simulink model "c6713dskfblms"  (Simulink 6.0)
settings: Solver=FixedStepDiscrete  StartTime=0.0  StopTime=inf  RelTol=1e-3
PreLoadFcn:
  | load handel; audiofrag = int16(y(1:2^16).*2^14); clear y;
undefined symbols (not defined in the file or in its folder): bit, FFT, FixedBlocks, Norm
libraries: tic62dsplib x17, dspmtrx3 x5, simulink x4, c6713dsklib x3, dspsnks4 x3, dspsigops x2, c6000tgtpreflib x1, dspbuff3 x1, dspxfrm3 x1, dspsrcs4 x1
settings Model: Creator=adowd  LastModifiedBy=thartley  ProdHWDeviceType=TI C6000
settings DataIOCC: SaveOutput=off  SaveTime=off  SignalLoggingName=sigsOut
settings OptimizationCC: InlineInvariantSignals=off  LocalBlockOutputs=off
settings DebuggingCC: CheckExecutionContextPreStartOutputMsg=on  CheckExecutionContextRuntimeOutputMsg=on  SolverPrmCheckMsg=none  IntegerOverflowMsg=none  ParameterPrecisionLossMsg=none
settings HardwareCC: ProdBitPerLong=40  ProdEndianess=LittleEndian  ProdHWDeviceType=TI C6000  TargetHWDeviceType=32-bit Generic
settings ModelReferenceCC: UpdateModelReferenceTargets=IfOutOfDate
settings RTWCC: SystemTargetFile=ti_c6000.tlc  GenCodeOnly=on  TemplateMakefile=ti_c6000.tmf  ProcessScript=ti_c6000_make_rtw_hook
settings CodeAppCC: PrefixModelToSubsysFcnNames=off
settings STFCustomTargetCC: TargetFcnLib=ansi_tfl_tmw.mat  GenFloatMathFcnCalls=ANSI_C  ModelReferenceCompliant=off  SystemTargetFile=ti_c6000.tlc  ActivateCallback=c6000_callback('ActivateCallback',hSrc,hDlg);  ForcedBaseTarget=off
settings GRTTargetCC: ModelReferenceCompliant=off  MatFileLogging=off
settings CustomProperty: DataType=RTWOptions_EnumType_s__Adsphw_matlab_toolbox_rtw_targets_tic6000_tic6000_ti_c6000_BoardType  Value=C6713DSK
settings EnumStrPairs: String=C6416DSK
settings SFSimCC: SFSimApplyToAllLibs=on  SFSimBuildMode=Incremental

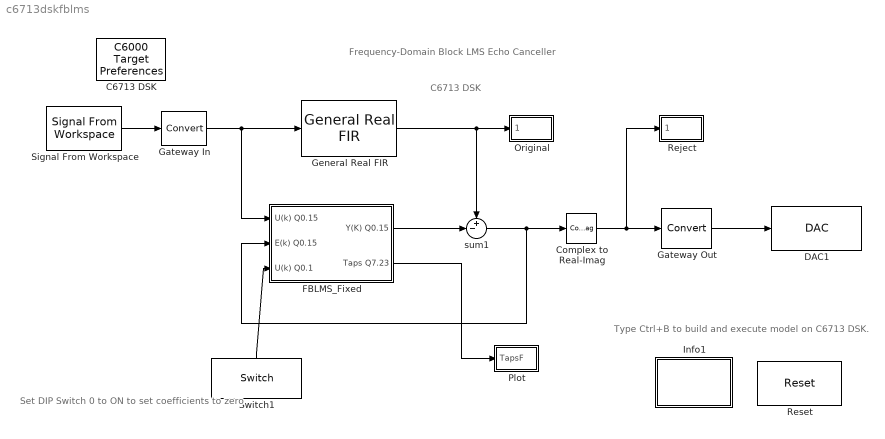
== system c6713dskfblms ==
  note: Frequency-Domain Block LMS
      | Echo Canceller
  note: Type Ctrl+B to build
      | and execute model
      | on C6713 DSK.
  note: C6713 DSK
  note: Set DIP Switch 0 to ON
      | to set coefficients to zero
  C6713 DSK : c6000tgtpreflib/C6000 Target Preferences
  Complex to Real-Imag : ComplexToRealImag  Output=Real
  DAC1 : c6713dsklib/DAC  CodecDataFormat=16-bit  Scaling=Integer Value  DacAtten=0.0  OverflowMode=Saturate
  FBLMS_Fixed : Subsystem  PropExecContextAcrossSSBoundary=on
  Gateway In : DataTypeConversion  OutDataTypeMode=Specify via dialog  OutDataType=sfrac(16)  OutScaling=2^-10  ConvertRealWorld=Stored Integer (SI)
  Gateway Out : DataTypeConversion  OutDataTypeMode=int16  ConvertRealWorld=Stored Integer (SI)
  General Real FIR : tic62dsplib/General Real FIR  coeff_source=Specify via dialog  coeffs=fir1(63,0.25)  ic_arg=0
  Info1 : Subsystem  PropExecContextAcrossSSBoundary=on
      settings: OpenFcn=web(fullfile(matlabroot,'toolbox','rtw','targets','tic6000','tic6000demos','html','fblms_doc.html'))
      mask Type: Frame-Based Simulation Info
      mask Display: disp('Info')
  Original : Subsystem  TreatAsAtomicUnit=on  PropExecContextAcrossSSBoundary=on  SimViewingDevice=on
  Plot : Subsystem  TreatAsAtomicUnit=on  PropExecContextAcrossSSBoundary=on  SimViewingDevice=on
  Reject : Subsystem  TreatAsAtomicUnit=on  PropExecContextAcrossSSBoundary=on  SimViewingDevice=on
  Reset : c6713dsklib/Reset
  Signal From Workspace : dspsrcs4/Signal From Workspace  X=audiofrag  Ts=1/8000  nsamps=64  OutputAfterFinalValue=Cyclic repetition
  Switch1 : c6713dsklib/Switch  Orientation=up  sw0=off  sw1=off  sw2=off  sw3=off  dType=Boolean  Ts=64/8000
  sum1 : Sum  Inputs=+-|  SaturateOnIntegerOverflow=on  InputSameDT=on
  wires:
  FBLMS_Fixed/1(Y(K) Q0.15) -> sum1/2
  General Real FIR/1 -> sum1/1, Original/1(Signal)
  Complex to Real-Imag/1 -> Gateway Out/1, Reject/1(Signal)
  Gateway Out/1 -> DAC1/1
  sum1/1 -> FBLMS_Fixed/2(E(k) Q0.15), Complex to Real-Imag/1
  Gateway In/1 -> General Real FIR/1, FBLMS_Fixed/1(U(k) Q0.15)
  FBLMS_Fixed/2(Taps Q7.23) -> Plot/1(TapsF)
  Signal From Workspace/1 -> Gateway In/1
  Switch1/1 -> FBLMS_Fixed/3(U(k) Q0.1)

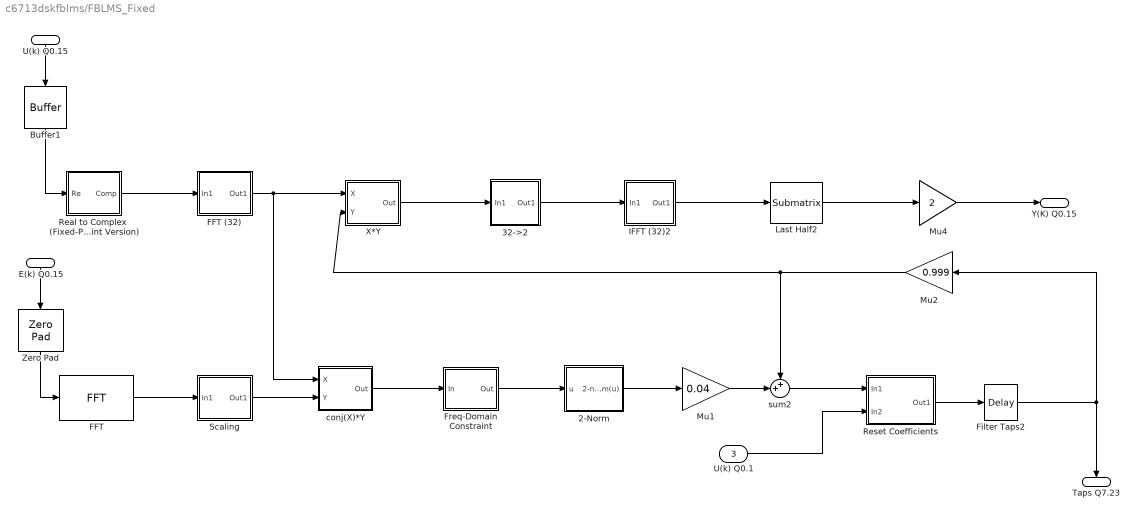
== system c6713dskfblms/FBLMS_Fixed ==
  U(k) Q0.15 : Inport  Orientation=down  LatchInput=off
  E(k) Q0.15 : Inport  Orientation=down  Port=2  LatchInput=off
  U(k) Q0.1 : Inport  Port=3  LatchInput=off
  2-Norm : Subsystem  AncestorBlock=FixedBlocks/2-Norm  PropExecContextAcrossSSBoundary=on
  32->2 : Subsystem  PropExecContextAcrossSSBoundary=on
  Buffer1 : dspbuff3/Buffer  Orientation=down  N=128  V=64  ic=0
  FFT : tic62dsplib/FFT
  FFT (32) : Subsystem  AncestorBlock=FixedBlocks/FFT (32)  PropExecContextAcrossSSBoundary=on  mask{nlen=128, prescale=1/4, postscale=32}
      mask prompts: nlen "Length (8 to 16384)"; prescale "Prescaling (8:32->1/4, 64:512->1/8)"; postscale "Postscaling"
      mask help:
      | This block performs an IFFT with output returned in normal (NOT bit-reversed order).
      | The implemented uses the FFT block.  This includes some scaling to avoid overflow
      | AND some scaling to compensate for scaling factors in FFT16X16R block
      mask CallbackString:
      | x = get_param(gcb,'MaskValues');
      | tscale = [2 2 4 4 8 8 16 16 32 32];
      | indx = round(log(eval(x{1}))/log(2)-2);
      | scale = tscale(indx);
      | x{3} = num2str(scale/eval(x{2}));
      | set_param(gcb,'MaskValues',x);|x = get_param(gcb,'MaskValues');
      | tscale = [2 2 4 4 8 8 16 16 32 32];
      | indx = round(log(eval(x{1}))/log(2)-2);
      | scale = tscale(indx);
      | x{3} = num2str(scale/eval(x{2}));
      | set_param(gcb,'MaskValues',x);|
  Filter Taps2 : dspsigops/Delay  dly_unit=Samples  delay=1  ic_detail=off  dif_ic_for_ch=off  dif_ic_for_dly=off  ic=0  reset_popup=None
  Freq-Domain Constraint : Subsystem  PropExecContextAcrossSSBoundary=on
  IFFT (32)2 : Subsystem  PropExecContextAcrossSSBoundary=on  mask{nlen=128, prescale=1/2, postscale=0.125}
      mask prompts: nlen "Length (8 to 16384)"; prescale "Prescaling"; postscale "Postscaling"
      mask init:
      | scale = 2.^(floor(log(nlen)/log(4))+1);
      | postscale = 1/(scale*prescale);
      mask CallbackString:
      | x = get_param(gcb,'MaskValues');
      | scale = 2.^(floor(log(eval(x{1}))/log(4))+1);
      | x{3} = num2str(1/(scale*eval(x{2})));
      | set_param(gcb,'MaskValues',x);|x = get_param(gcb,'MaskValues');
      | scale = 2.^(floor(log(eval(x{1}))/log(4))+1);
      | x{3} = num2str(1/(scale*eval(x{2})));
      | set_param(gcb,'MaskValues',x);|
  Last Half2 : dspmtrx3/Submatrix  RowSpan=Range of rows  RowStartMode=Offset from middle  RowStartIndex=0  RowEndMode=Last  RowEndIndex=L  ColSpan=All columns  ColStartMode=First  ColStartIndex=1  ColEndMode=Last  ColEndIndex=1
  Mu1 : Gain  Gain=0.04  OutDataTypeMode=Specify via dialog  OutDataType=sfix(32)  OutScaling=2^-31
  Mu2 : Gain  Orientation=left  Gain=0.999  SaturateOnIntegerOverflow=on
  Mu4 : Gain  Gain=2  SaturateOnIntegerOverflow=on
  Real to Complex  (Fixed-Point Version) : Subsystem  PropExecContextAcrossSSBoundary=on
  Reset Coefficients : Subsystem  PropExecContextAcrossSSBoundary=on
  Scaling : Subsystem  PropExecContextAcrossSSBoundary=on
  X*Y : Subsystem  PropExecContextAcrossSSBoundary=on
  Zero Pad : dspsigops/Zero Pad  Orientation=down  padSigAt=Beginning  zpadAlong=Columns  padNumOutRowsSpecMethod=User-specified  numOutRows=128  padNumOutColsSpecMethod=Next power of two  numOutCols=1  trunc_flag=None
      settings: AttributesFormatString=\n
  conj(X)*Y : Subsystem  PropExecContextAcrossSSBoundary=on
  sum2 : Sum  Inputs=++|  OutDataTypeMode=Specify via dialog  OutDataType=sfix(32)  OutScaling=2^-24  SaturateOnIntegerOverflow=on
  Y(K) Q0.15 : Outport
  Taps Q7.23 : Outport  Orientation=down  Port=2
  wires:
  U(k) Q0.15/1 -> Buffer1/1
  Buffer1/1 -> Real to Complex  (Fixed-Point Version)/1(Re)
  Zero Pad/1 -> FFT/1
  FFT (32)/1(Out1) -> X*Y/1(X), conj(X)*Y/1(X)
  FFT/1 -> Scaling/1(In1)
  conj(X)*Y/1(Out) -> Freq-Domain Constraint/1(In)
  Filter Taps2/1 -> Mu2/1, Taps Q7.23/1
  X*Y/1(Out) -> 32->2/1(In1)
  IFFT (32)2/1(Out1) -> Last Half2/1
  32->2/1(Out1) -> IFFT (32)2/1(In1)
  Last Half2/1 -> Mu4/1
  Mu1/1 -> sum2/2
  Mu4/1 -> Y(K) Q0.15/1
  Scaling/1(Out1) -> conj(X)*Y/2(Y)
  Real to Complex  (Fixed-Point Version)/1(Comp) -> FFT (32)/1(In1)
  E(k) Q0.15/1 -> Zero Pad/1
  Freq-Domain Constraint/1(Out) -> 2-Norm/1(u)
  2-Norm/1(2-norm(u)) -> Mu1/1
  Reset Coefficients/1(Out1) -> Filter Taps2/1
  U(k) Q0.1/1 -> Reset Coefficients/2(In2)
  Mu2/1 -> sum2/1, X*Y/2(Y)
  sum2/1 -> Reset Coefficients/1(In1)

== system c6713dskfblms/Info1 ==

== system c6713dskfblms/Original ==
  Signal : Inport  LatchInput=off
  Gateway Out1 : DataTypeConversion  OutDataTypeMode=double
  Original : dspsnks4/Vector Scope  ScopeProperties=off  Domain=Time  HorizSpan=10  DisplayProperties=on  AxisGrid=on  Memory=off  FrameNumber=on  AxisLegend=off  AxisZoom=off  OpenScopeAtSimStart=on  OpenScopeImmediately=off  FigPos=[89 447 428 214]  AxisProperties=off  XUnits=Hertz  XRange=[0...Fs/2]  InheritXIncr=on  XIncr=1  XLabel=Time  YUnits=dB  YLabel=Amplitude  LineProperties=off
      settings: AttributesFormatString=\n\n  YMin=-0.35  YMax=0.35
  wires:
  Gateway Out1/1 -> Original/1
  Signal/1 -> Gateway Out1/1

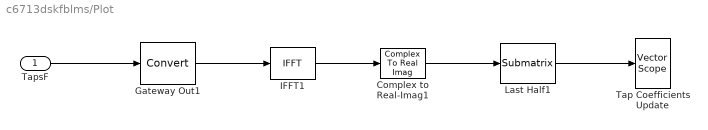
== system c6713dskfblms/Plot ==
  TapsF : Inport  LatchInput=off
  Complex to Real-Imag1 : ComplexToRealImag  Output=Real
  Gateway Out1 : DataTypeConversion  OutDataTypeMode=double
  IFFT1 : dspxfrm3/IFFT  DialogController=dspDDGCreate  DialogControllerArgs=DataTag1  CompMethod=Table lookup  TableOpt=Speed  BitRevOrder=off  cs_in=off  SkipNorm=off  mode=Real  firstCoeffMode=User-defined  firstCoeffWordLength=16  firstCoeffFracLength=15  roundingMode=Floor  overflowMode=off
  Last Half1 : dspmtrx3/Submatrix  RowSpan=Range of rows  RowStartMode=Index  RowStartIndex=1  RowEndMode=Middle  RowEndIndex=1  ColSpan=All columns  ColStartMode=First  ColStartIndex=1  ColEndMode=Last  ColEndIndex=1
  "Tap Coefficients Update " : dspsnks4/Vector Scope  ScopeProperties=off  Domain=Time  HorizSpan=1  DisplayProperties=on  AxisGrid=on  Memory=off  FrameNumber=on  AxisLegend=off  AxisZoom=off  OpenScopeAtSimStart=on  OpenScopeImmediately=off  FigPos=[524 447 428 214]  AxisProperties=off  XUnits=Hertz  XRange=[0...Fs/2]  InheritXIncr=on  XIncr=1  XLabel=Time  YUnits=dB  YLabel=Amplitude  LineProperties=off
      settings: AttributesFormatString=\n\n  YMin=-1.1  YMax=3
  wires:
  IFFT1/1 -> Complex to Real-Imag1/1
  Complex to Real-Imag1/1 -> Last Half1/1
  Gateway Out1/1 -> IFFT1/1
  Last Half1/1 -> "Tap Coefficients Update "/1
  TapsF/1 -> Gateway Out1/1

== system c6713dskfblms/Reject ==
  Signal : Inport  LatchInput=off
  Gateway Out1 : DataTypeConversion  OutDataTypeMode=double
  Reject : dspsnks4/Vector Scope  ScopeProperties=off  Domain=Time  HorizSpan=10  DisplayProperties=on  AxisGrid=on  Memory=off  FrameNumber=on  AxisLegend=off  AxisZoom=off  OpenScopeAtSimStart=on  OpenScopeImmediately=off  FigPos=[88 183 428 219]  AxisProperties=off  XUnits=Hertz  XRange=[0...Fs/2]  InheritXIncr=on  XIncr=1  XLabel=Time  YUnits=dB  YLabel=Amplitude  LineProperties=off
      settings: AttributesFormatString=\n\n  YMin=-0.35  YMax=0.35
  wires:
  Gateway Out1/1 -> Reject/1
  Signal/1 -> Gateway Out1/1

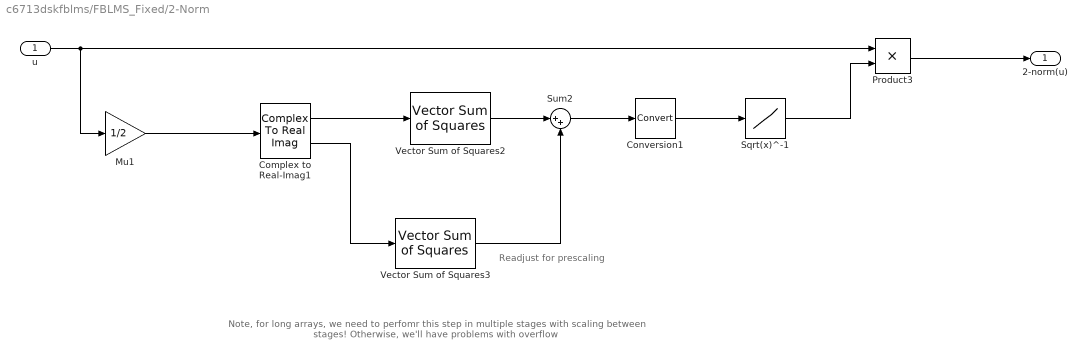
== system c6713dskfblms/FBLMS_Fixed/2-Norm ==
  note: Note, for long arrays, we need to
      | perfomr this step in multiple stages
      | with scaling between stages!
      | Otherwise, we'll have problems with
      | overflow
  note: Readjust for prescaling
  u : Inport  LatchInput=off
  Complex to Real-Imag1 : ComplexToRealImag
  Conversion1 : DataTypeConversion  OutDataTypeMode=Specify via dialog  OutDataType=ufix(16)  OutScaling=2^-13  SaturateOnIntegerOverflow=on
  Mu1 : Gain  Gain=1/2  OutDataType=sfix(32)  OutScaling=2^-31
  Product3 : Product  OutDataType=sfix(32)  OutScaling=2^30  SaturateOnIntegerOverflow=on
  Sqrt(x)^-1 : Lookup  DialogController=Simulink.DDGSource  InputValues=[0.004 0.01 linspace(0.02,8,62)]  OutputValues=1./sqrt([0.004 0.01 linspace(0.02,8,62)])  LookUpMeth=Use Input Nearest  OutDataTypeMode=Specify via dialog  OutDataType=ufix(16)  OutScaling=2^-12  SaturateOnIntegerOverflow=on
  Sum2 : Sum  Inputs=|++  OutDataType=ufix(16)  OutScaling=2^14  SaturateOnIntegerOverflow=on
  Vector Sum of Squares2 : tic62dsplib/Vector Sum of Squares
  Vector Sum of Squares3 : tic62dsplib/Vector Sum of Squares
  2-norm(u) : Outport
  wires:
  Product3/1 -> 2-norm(u)/1
  Sqrt(x)^-1/1 -> Product3/2
  Complex to Real-Imag1/2 -> Vector Sum of Squares3/1
  Vector Sum of Squares2/1 -> Sum2/1
  Vector Sum of Squares3/1 -> Sum2/2
  Sum2/1 -> Conversion1/1
  Complex to Real-Imag1/1 -> Vector Sum of Squares2/1
  Conversion1/1 -> Sqrt(x)^-1/1
  Mu1/1 -> Complex to Real-Imag1/1
  u/1 -> Mu1/1, Product3/1

== system c6713dskfblms/FBLMS_Fixed/32->2 ==
  In1 : Inport  LatchInput=off
  Conversion : DataTypeConversion  OutDataTypeMode=Specify via dialog  OutScaling=2^-10  SaturateOnIntegerOverflow=on
  Conversion1 : DataTypeConversion  OutDataTypeMode=Specify via dialog  OutDataType=sfrac(16)  OutScaling=2^-7  ConvertRealWorld=Stored Integer (SI)
  Out1 : Outport
  wires:
  Conversion1/1 -> Out1/1
  In1/1 -> Conversion/1
  Conversion/1 -> Conversion1/1

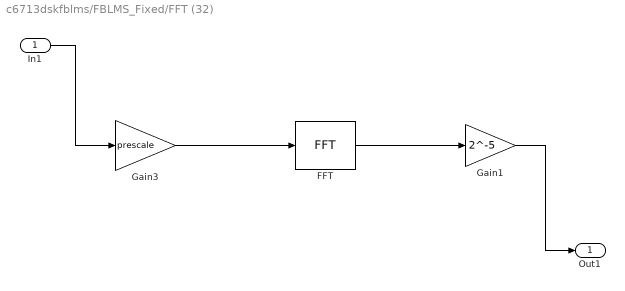
== system c6713dskfblms/FBLMS_Fixed/FFT (32) ==
  In1 : Inport  LatchInput=off
  FFT : tic62dsplib/FFT
  Gain1 : Gain  Gain=2^-5  ParameterDataTypeMode=Specify via dialog  SaturateOnIntegerOverflow=on
  Gain3 : Gain  Gain=prescale  SaturateOnIntegerOverflow=on
  Out1 : Outport
  wires:
  FFT/1 -> Gain1/1
  In1/1 -> Gain3/1
  Gain3/1 -> FFT/1
  Gain1/1 -> Out1/1

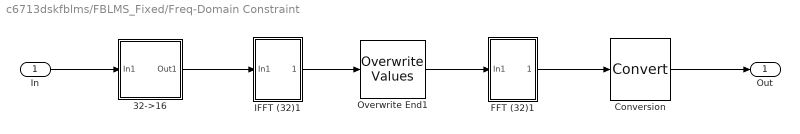
== system c6713dskfblms/FBLMS_Fixed/Freq-Domain Constraint ==
  In : Inport  LatchInput=off
  32->16 : Subsystem  PropExecContextAcrossSSBoundary=on
  Conversion : DataTypeConversion  OutDataTypeMode=Specify via dialog  OutScaling=2^-14
  FFT (32)1 : Subsystem  PropExecContextAcrossSSBoundary=on  mask{nlen=128, prescale=1/4, postscale=32}
      mask prompts: nlen "Length (8 to 16384)"; prescale "Prescaling (8:32->1/4, 64:512->1/8)"; postscale "Postscaling"
      mask help:
      | This block performs an IFFT with output returned in normal (NOT bit-reversed order).
      | The implemented uses the FFT block.  This includes some scaling to avoid overflow
      | AND some scaling to compensate for scaling factors in FFT16X16R block
      mask CallbackString:
      | x = get_param(gcb,'MaskValues');
      | tscale = [2 2 4 4 8 8 16 16 32 32];
      | indx = round(log(eval(x{1}))/log(2)-2);
      | scale = tscale(indx);
      | x{3} = num2str(scale/eval(x{2}));
      | set_param(gcb,'MaskValues',x);|x = get_param(gcb,'MaskValues');
      | tscale = [2 2 4 4 8 8 16 16 32 32];
      | indx = round(log(eval(x{1}))/log(2)-2);
      | scale = tscale(indx);
      | x{3} = num2str(scale/eval(x{2}));
      | set_param(gcb,'MaskValues',x);|
  IFFT (32)1 : Subsystem  PropExecContextAcrossSSBoundary=on  mask{nlen=128, prescale=1/2, postscale=0.125}
      mask prompts: nlen "Length (8 to 16384)"; prescale "Prescaling"; postscale "Postscaling"
      mask init:
      | scale = 2.^(floor(log(nlen)/log(4))+1);
      | postscale = 1/(scale*prescale);
      mask CallbackString:
      | x = get_param(gcb,'MaskValues');
      | scale = 2.^(floor(log(eval(x{1}))/log(4))+1);
      | x{3} = num2str(1/(scale*eval(x{2})));
      | set_param(gcb,'MaskValues',x);|x = get_param(gcb,'MaskValues');
      | scale = 2.^(floor(log(eval(x{1}))/log(4))+1);
      | x{3} = num2str(1/(scale*eval(x{2})));
      | set_param(gcb,'MaskValues',x);|
  Overwrite End1 : dspmtrx3/Overwrite Values  OverWriteDiag=Submatrix  valFrom2ndIP=Specify via dialog  ConstValue=0  RowSpan=Range of rows  RowStartMode=Middle  RowStartIndex=1  RowEndMode=Last  RowEndIndex=-1  ColSpan=All columns  ColStartMode=First  ColStartIndex=1  ColEndMode=Last  ColEndIndex=1  DiagSpan=Range of elements  DiagStartMode=Index  DiagStartIndex=2  DiagEndMode=Index  DiagEndIndex=4
      settings: AttributesFormatString=\n
  Out : Outport
  wires:
  IFFT (32)1/1(Out1) -> Overwrite End1/1
  Overwrite End1/1 -> FFT (32)1/1(In1)
  FFT (32)1/1(Out1) -> Conversion/1
  32->16/1(Out1) -> IFFT (32)1/1(In1)
  In/1 -> 32->16/1(In1)
  Conversion/1 -> Out/1

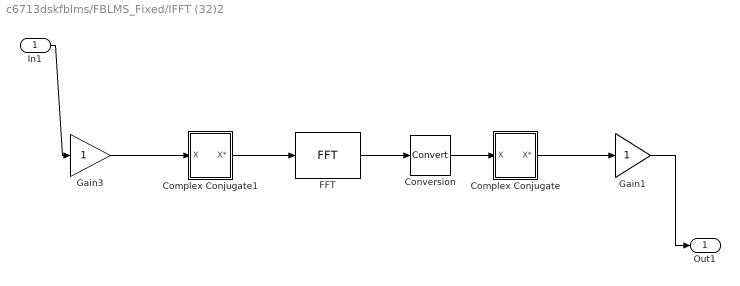
== system c6713dskfblms/FBLMS_Fixed/IFFT (32)2 ==
  In1 : Inport  LatchInput=off
  Complex Conjugate : Subsystem  PropExecContextAcrossSSBoundary=on
  Complex Conjugate1 : Subsystem  PropExecContextAcrossSSBoundary=on
  Conversion : DataTypeConversion  OutDataTypeMode=Specify via dialog  OutScaling=2^-15
  FFT : tic62dsplib/FFT
  Gain1 : Gain  SaturateOnIntegerOverflow=on
  Gain3 : Gain  SaturateOnIntegerOverflow=on
  Out1 : Outport
  wires:
  Gain1/1 -> Out1/1
  Gain3/1 -> Complex Conjugate1/1(X)
  Complex Conjugate/1(X*) -> Gain1/1
  In1/1 -> Gain3/1
  FFT/1 -> Conversion/1
  Complex Conjugate1/1(X*) -> FFT/1
  Conversion/1 -> Complex Conjugate/1(X)

== system c6713dskfblms/FBLMS_Fixed/Real to Complex  (Fixed-Point Version) ==
  Re : Inport  Orientation=up  LatchInput=off
  Overwrite End2 : dspmtrx3/Overwrite Values  OverWriteDiag=Submatrix  valFrom2ndIP=Specify via dialog  ConstValue=0  RowSpan=Range of rows  RowStartMode=First  RowStartIndex=1  RowEndMode=Last  RowEndIndex=-1  ColSpan=All columns  ColStartMode=First  ColStartIndex=1  ColEndMode=Last  ColEndIndex=1  DiagSpan=Range of elements  DiagStartMode=Index  DiagStartIndex=2  DiagEndMode=Index  DiagEndIndex=4
      settings: AttributesFormatString=\n
  Real-Imag to Complex1 : RealImagToComplex
  Comp : Outport
  wires:
  Real-Imag to Complex1/1 -> Comp/1
  Overwrite End2/1 -> Real-Imag to Complex1/2
  Re/1 -> Real-Imag to Complex1/1, Overwrite End2/1

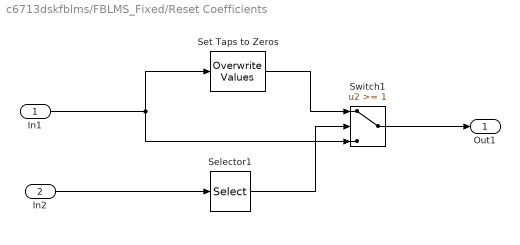
== system c6713dskfblms/FBLMS_Fixed/Reset Coefficients ==
  In1 : Inport  LatchInput=off
  In2 : Inport  Port=2  LatchInput=off
  Selector1 : Selector  InputPortWidth=4
  Set Taps to Zeros : dspmtrx3/Overwrite Values  OverWriteDiag=Submatrix  valFrom2ndIP=Specify via dialog  ConstValue=0  RowSpan=All rows  RowStartMode=Middle  RowStartIndex=1  RowEndMode=Last  RowEndIndex=-1  ColSpan=All columns  ColStartMode=First  ColStartIndex=1  ColEndMode=Last  ColEndIndex=1  DiagSpan=Range of elements  DiagStartMode=Index  DiagStartIndex=2  DiagEndMode=Index  DiagEndIndex=4
      settings: AttributesFormatString=\n
  Switch1 : Switch  Threshold=1  ZeroCross=off  InputSameDT=on
  Out1 : Outport
  wires:
  Selector1/1 -> Switch1/2
  In1/1 -> Set Taps to Zeros/1, Switch1/3
  Set Taps to Zeros/1 -> Switch1/1
  Switch1/1 -> Out1/1
  In2/1 -> Selector1/1

== system c6713dskfblms/FBLMS_Fixed/Scaling ==
  In1 : Inport  LatchInput=off
  Conversion1 : DataTypeConversion  OutDataTypeMode=Specify via dialog  OutDataType=sfix(32)  OutScaling=2^-24
  Mu5 : Gain  Gain=8  OutDataType=sfix(32)  SaturateOnIntegerOverflow=on
  Out1 : Outport
  wires:
  Conversion1/1 -> Mu5/1
  In1/1 -> Conversion1/1
  Mu5/1 -> Out1/1

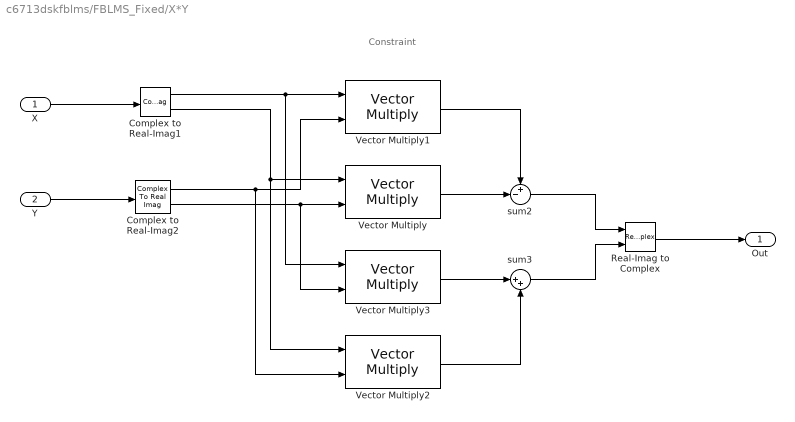
== system c6713dskfblms/FBLMS_Fixed/X*Y ==
  note: Constraint
  X : Inport  LatchInput=off
  Y : Inport  Port=2  LatchInput=off
  Complex to Real-Imag1 : ComplexToRealImag
  Complex to Real-Imag2 : ComplexToRealImag
  Real-Imag to Complex : RealImagToComplex
  Vector Multiply{,1..3} (4 alike) : tic62dsplib/Vector Multiply
  sum2 : Sum  Inputs=+-|  OutDataType=sfrac(16)  SaturateOnIntegerOverflow=on  InputSameDT=on
  sum3 : Sum  Inputs=|++  OutDataType=sfrac(16)  SaturateOnIntegerOverflow=on  InputSameDT=on
  Out : Outport
  wires:
  Real-Imag to Complex/1 -> Out/1
  Y/1 -> Complex to Real-Imag2/1
  X/1 -> Complex to Real-Imag1/1
  Vector Multiply1/1 -> sum2/1
  Vector Multiply/1 -> sum2/2
  sum3/1 -> Real-Imag to Complex/2
  Vector Multiply2/1 -> sum3/2
  Vector Multiply3/1 -> sum3/1
  sum2/1 -> Real-Imag to Complex/1
  Complex to Real-Imag1/1 -> Vector Multiply3/1, Vector Multiply1/1
  Complex to Real-Imag2/1 -> Vector Multiply2/2, Vector Multiply1/2
  Complex to Real-Imag1/2 -> Vector Multiply2/1, Vector Multiply/1
  Complex to Real-Imag2/2 -> Vector Multiply/2, Vector Multiply3/2

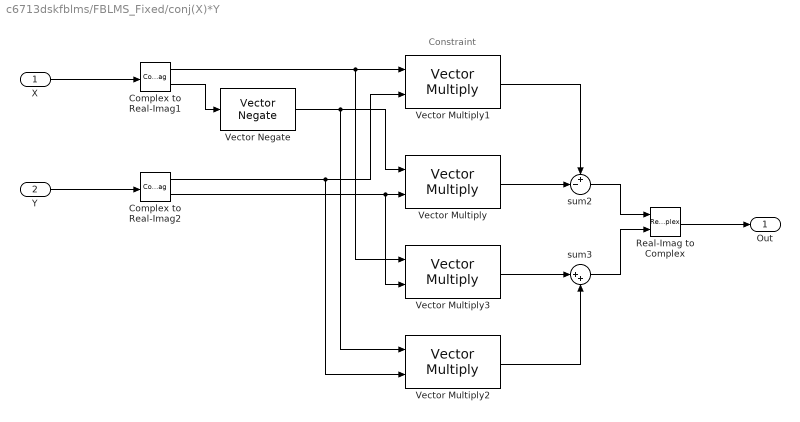
== system c6713dskfblms/FBLMS_Fixed/conj(X)*Y ==
  note: Constraint
  X : Inport  LatchInput=off
  Y : Inport  Port=2  LatchInput=off
  Complex to Real-Imag1 : ComplexToRealImag
  Complex to Real-Imag2 : ComplexToRealImag
  Real-Imag to Complex : RealImagToComplex
  Vector Multiply{,1..3} (4 alike) : tic62dsplib/Vector Multiply
  Vector Negate : tic62dsplib/Vector Negate
  sum2 : Sum  Inputs=+-|  OutDataType=sfrac(16)  SaturateOnIntegerOverflow=on  InputSameDT=on
  sum3 : Sum  Inputs=|++  OutDataType=sfrac(16)  SaturateOnIntegerOverflow=on  InputSameDT=on
  Out : Outport
  wires:
  Complex to Real-Imag1/2 -> Vector Negate/1
  Vector Negate/1 -> Vector Multiply/1, Vector Multiply2/1
  Complex to Real-Imag2/2 -> Vector Multiply/2, Vector Multiply3/2
  Complex to Real-Imag2/1 -> Vector Multiply1/2, Vector Multiply2/2
  Complex to Real-Imag1/1 -> Vector Multiply1/1, Vector Multiply3/1
  Vector Multiply3/1 -> sum3/1
  Vector Multiply2/1 -> sum3/2
  sum3/1 -> Real-Imag to Complex/2
  Vector Multiply/1 -> sum2/2
  Vector Multiply1/1 -> sum2/1
  X/1 -> Complex to Real-Imag1/1
  Y/1 -> Complex to Real-Imag2/1
  Real-Imag to Complex/1 -> Out/1
  sum2/1 -> Real-Imag to Complex/1

== system c6713dskfblms/FBLMS_Fixed/Freq-Domain Constraint/32->16 ==
  In1 : Inport  LatchInput=off
  Conversion : DataTypeConversion  OutDataTypeMode=Specify via dialog  OutScaling=2^-9  RndMeth=Nearest  SaturateOnIntegerOverflow=on
  Conversion1 : DataTypeConversion  OutDataTypeMode=Specify via dialog  OutDataType=sfrac(16)  OutScaling=2^-7  ConvertRealWorld=Stored Integer (SI)
  Out1 : Outport
  wires:
  Conversion/1 -> Conversion1/1
  In1/1 -> Conversion/1
  Conversion1/1 -> Out1/1

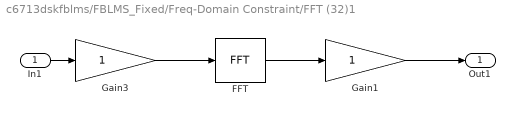
== system c6713dskfblms/FBLMS_Fixed/Freq-Domain Constraint/FFT (32)1 ==
  In1 : Inport  LatchInput=off
  FFT : tic62dsplib/FFT
  Gain1 : Gain  ParameterDataTypeMode=Specify via dialog  SaturateOnIntegerOverflow=on
  Gain3 : Gain  SaturateOnIntegerOverflow=on
  Out1 : Outport
  wires:
  FFT/1 -> Gain1/1
  In1/1 -> Gain3/1
  Gain3/1 -> FFT/1
  Gain1/1 -> Out1/1

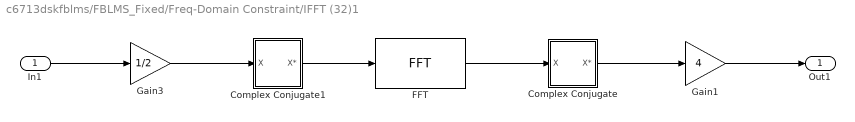
== system c6713dskfblms/FBLMS_Fixed/Freq-Domain Constraint/IFFT (32)1 ==
  In1 : Inport  LatchInput=off
  Complex Conjugate : Subsystem  PropExecContextAcrossSSBoundary=on
  Complex Conjugate1 : Subsystem  PropExecContextAcrossSSBoundary=on
  FFT : tic62dsplib/FFT
  Gain1 : Gain  Gain=4  SaturateOnIntegerOverflow=on
  Gain3 : Gain  Gain=1/2  SaturateOnIntegerOverflow=on
  Out1 : Outport
  wires:
  Gain1/1 -> Out1/1
  Gain3/1 -> Complex Conjugate1/1(X)
  Complex Conjugate/1(X*) -> Gain1/1
  In1/1 -> Gain3/1
  FFT/1 -> Complex Conjugate/1(X)
  Complex Conjugate1/1(X*) -> FFT/1

== system c6713dskfblms/FBLMS_Fixed/IFFT (32)2/Complex Conjugate ==
  X : Inport  LatchInput=off
  Complex to Real-Imag : ComplexToRealImag
  Real-Imag to Complex : RealImagToComplex
  Unary Minus : simulink/Math Operations/Unary Minus  DoSatur=off
  X* : Outport
  wires:
  Complex to Real-Imag/2 -> Unary Minus/1
  Unary Minus/1 -> Real-Imag to Complex/2
  Complex to Real-Imag/1 -> Real-Imag to Complex/1
  X/1 -> Complex to Real-Imag/1
  Real-Imag to Complex/1 -> X*/1

== system c6713dskfblms/FBLMS_Fixed/IFFT (32)2/Complex Conjugate1 ==
  X : Inport  LatchInput=off
  Complex to Real-Imag : ComplexToRealImag
  Real-Imag to Complex : RealImagToComplex
  Unary Minus : simulink/Math Operations/Unary Minus  DoSatur=off
  X* : Outport
  wires:
  Complex to Real-Imag/2 -> Unary Minus/1
  Unary Minus/1 -> Real-Imag to Complex/2
  Complex to Real-Imag/1 -> Real-Imag to Complex/1
  X/1 -> Complex to Real-Imag/1
  Real-Imag to Complex/1 -> X*/1

== system c6713dskfblms/FBLMS_Fixed/Freq-Domain Constraint/IFFT (32)1/Complex Conjugate ==
  X : Inport  LatchInput=off
  Complex to Real-Imag : ComplexToRealImag
  Real-Imag to Complex : RealImagToComplex
  Unary Minus : simulink/Math Operations/Unary Minus  DoSatur=off
  X* : Outport
  wires:
  Complex to Real-Imag/2 -> Unary Minus/1
  Unary Minus/1 -> Real-Imag to Complex/2
  Complex to Real-Imag/1 -> Real-Imag to Complex/1
  X/1 -> Complex to Real-Imag/1
  Real-Imag to Complex/1 -> X*/1

== system c6713dskfblms/FBLMS_Fixed/Freq-Domain Constraint/IFFT (32)1/Complex Conjugate1 ==
  X : Inport  LatchInput=off
  Complex to Real-Imag : ComplexToRealImag
  Real-Imag to Complex : RealImagToComplex
  Unary Minus : simulink/Math Operations/Unary Minus  DoSatur=off
  X* : Outport
  wires:
  Complex to Real-Imag/2 -> Unary Minus/1
  Unary Minus/1 -> Real-Imag to Complex/2
  Complex to Real-Imag/1 -> Real-Imag to Complex/1
  X/1 -> Complex to Real-Imag/1
  Real-Imag to Complex/1 -> X*/1
